simulink model "FSTABSMC"  (R2024b)
settings: Solver=VariableStepAuto  StartTime=0.0  StopTime=20  RelTol=1e-3
settings Model: Creator=amlak  LastModifiedBy=amlak

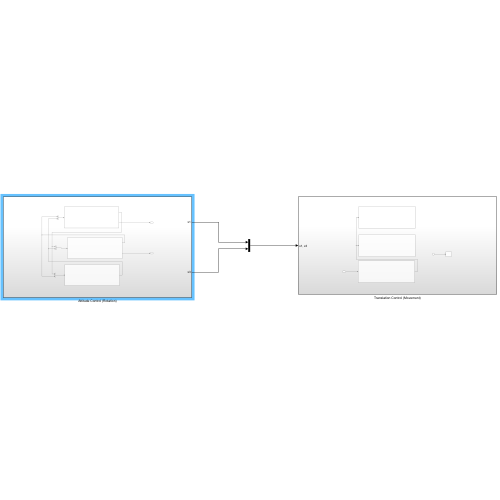
[thumbnail: Simulink's stored preview of the top-level diagram]
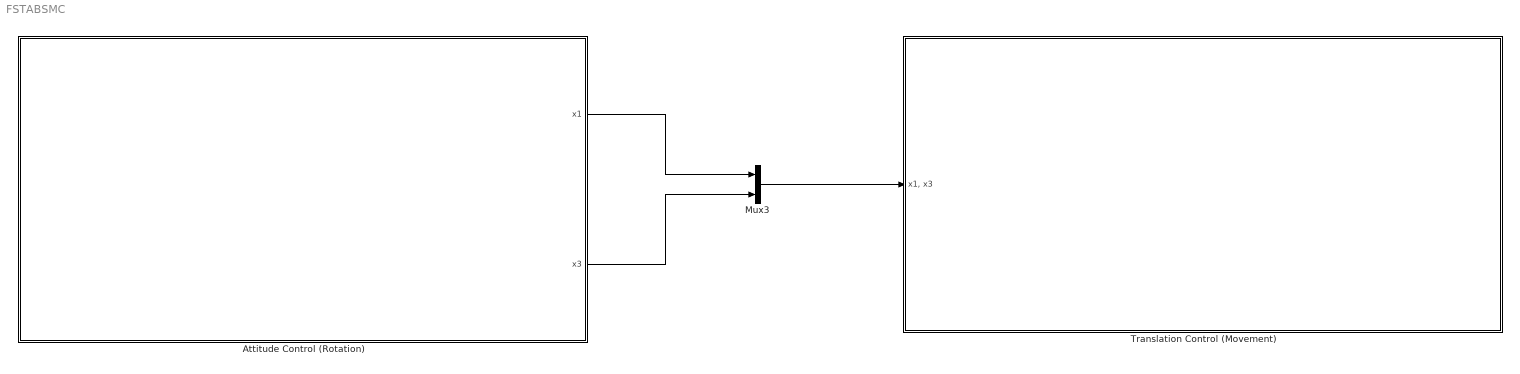
== system FSTABSMC ==
  Attitude Control (Rotation) : Subsystem
  Mux3 : Mux  Inputs=2
  Translation Control (Movement) : Subsystem
  wires:
  Attitude Control (Rotation)/1(x1) -> Mux3/1
  Attitude Control (Rotation)/2(x3) -> Mux3/2
  Mux3/1 -> Translation Control (Movement)/1("x1, x3")

== system FSTABSMC/Attitude Control (Rotation) ==
  Mux : Mux  Inputs=2
  Mux1 : Mux  Inputs=2
  Mux2 : Mux  Inputs=2
  PITCH Controller : Subsystem
  "ROLL Controller " : Subsystem
  YAW Controller : Subsystem
  x1 : Outport
  x3 : Outport  Port=2
  wires:
  YAW Controller/1(x6) -> Mux1/2, Mux/2
  PITCH Controller/1(x4) -> Mux/1, Mux2/2
  "ROLL Controller "/1(x2) -> Mux2/1, Mux1/1
  PITCH Controller/2(x3) -> x3/1
  Mux1/1 -> PITCH Controller/1(In1)
  Mux2/1 -> YAW Controller/1(In1)
  Mux/1 -> "ROLL Controller "/1(In1)
  "ROLL Controller "/2(x1) -> x1/1

== system FSTABSMC/Translation Control (Movement) ==
  "x1, x3" : Inport
  Clock : Clock
      settings: Decimation=20
  To Workspace1 : ToWorkspace  VariableName=t  SampleTime=-1
      settings: Save2DSignal=2-D array (concatenate along first dimension)
  X Trajectory Controller : Subsystem
  Y Trajectory Controller : Subsystem
  "Z Trajectory Controller " : Subsystem
  wires:
  "Z Trajectory Controller "/1(U1) -> X Trajectory Controller/1(U1), Y Trajectory Controller/1(U1)
  "x1, x3"/1 -> "Z Trajectory Controller "/1("x1, x3")
  Clock/1 -> To Workspace1/1

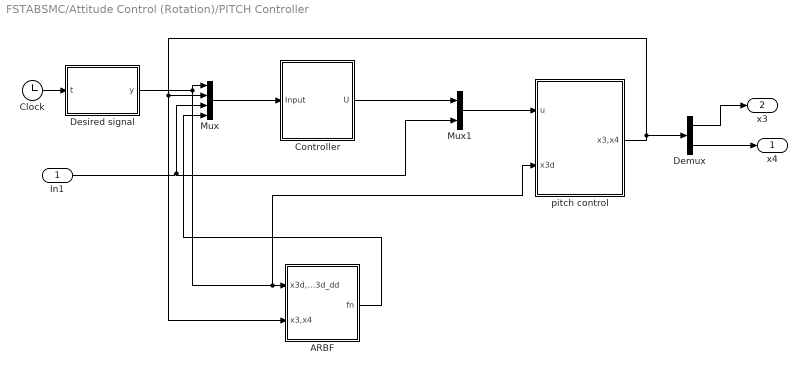
== system FSTABSMC/Attitude Control (Rotation)/PITCH Controller ==
  In1 : Inport
  ARBF : Subsystem
  Clock : Clock
      settings: Decimation=20
  Controller : Subsystem
  Demux : Demux  Outputs=2
  Desired signal : MATLAB Function  TreatAsAtomicUnit=on
  Mux : Mux
  Mux1 : Mux  Inputs=2
  pitch control : Subsystem
  x4 : Outport
  x3 : Outport  Port=2
  wires:
  Desired signal/1(y) -> pitch control/2(x3d), ARBF/1("x3d, x3d_dot, x3d_dd"), Mux/1
  Clock/1 -> Desired signal/1(t)
  pitch control/1(x3,x4) -> Demux/1, ARBF/2(x3,x4), Mux/2
  In1/1 -> Mux/3, Mux1/2
  Mux/1 -> Controller/1(Input)
  Controller/1(U) -> Mux1/1
  Mux1/1 -> pitch control/1(u)
  ARBF/1(fn) -> Mux/4
  Demux/2 -> x4/1
  Demux/1 -> x3/1

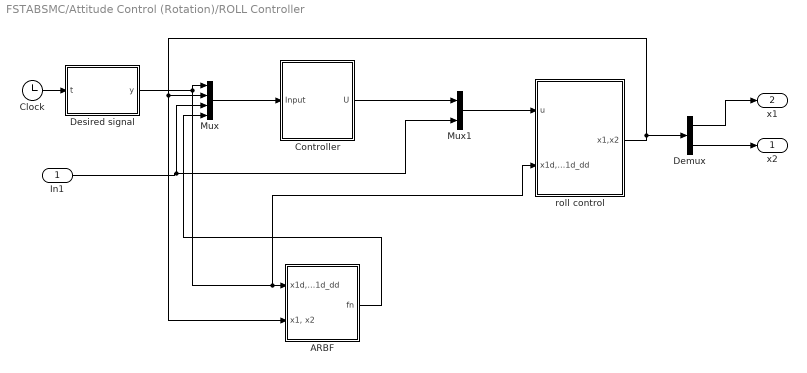
== system FSTABSMC/Attitude Control (Rotation)/ROLL Controller  ==
  In1 : Inport
  ARBF : Subsystem
  Clock : Clock
      settings: Decimation=20
  Controller : Subsystem
  Demux : Demux  Outputs=2
  Desired signal : MATLAB Function  TreatAsAtomicUnit=on
  Mux : Mux
  Mux1 : Mux  Inputs=2
  roll control : Subsystem
  x2 : Outport
  x1 : Outport  Port=2
  wires:
  Desired signal/1(y) -> roll control/2("x1d, x1d_d, x1d_dd"), ARBF/1("x1d, x1d_d, x1d_dd"), Mux/1
  Clock/1 -> Desired signal/1(t)
  roll control/1(x1,x2) -> Demux/1, ARBF/2("x1, x2"), Mux/2
  In1/1 -> Mux1/2, Mux/3
  Mux/1 -> Controller/1(Input)
  Controller/1(U) -> Mux1/1
  Mux1/1 -> roll control/1(u)
  ARBF/1(fn) -> Mux/4
  Demux/2 -> x2/1
  Demux/1 -> x1/1

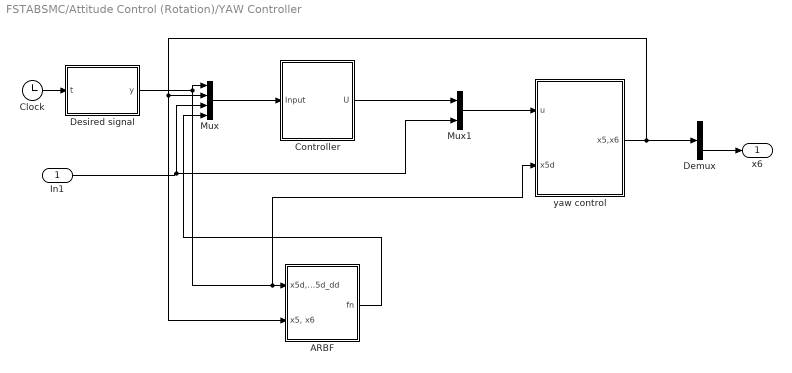
== system FSTABSMC/Attitude Control (Rotation)/YAW Controller ==
  In1 : Inport
  ARBF : Subsystem
  Clock : Clock
      settings: Decimation=20
  Controller : Subsystem
  Demux : Demux  Outputs=2
  Desired signal : MATLAB Function  TreatAsAtomicUnit=on
  Mux : Mux
  Mux1 : Mux  Inputs=2
  yaw control : Subsystem
  x6 : Outport
  wires:
  Desired signal/1(y) -> yaw control/2(x5d), ARBF/1("x5d, x5d_d, x5d_dd"), Mux/1
  Clock/1 -> Desired signal/1(t)
  yaw control/1(x5,x6) -> Demux/1, ARBF/2("x5, x6"), Mux/2
  In1/1 -> Mux1/2, Mux/3
  Mux/1 -> Controller/1(Input)
  Controller/1(U) -> Mux1/1
  Mux1/1 -> yaw control/1(u)
  ARBF/1(fn) -> Mux/4
  Demux/2 -> x6/1

== system FSTABSMC/Translation Control (Movement)/X Trajectory Controller ==
  U1 : Inport
  ARBF : Subsystem
  Clock : Clock
      settings: Decimation=20
  Controller : Subsystem
  Desired signal : MATLAB Function  TreatAsAtomicUnit=on
  Mux : Mux
  Mux1 : Mux  Inputs=2
  x-axis control : Subsystem
  wires:
  Desired signal/1(y) -> x-axis control/2(x7d), ARBF/1("x7d, x7d_d, x7d_dd"), Mux/1
  Clock/1 -> Desired signal/1(t)
  x-axis control/1("x7, x8") -> ARBF/2(x7,x8), Mux/2
  U1/1 -> Mux1/2, Mux/3
  Mux/1 -> Controller/1(Input)
  Controller/1(U) -> Mux1/1
  Mux1/1 -> x-axis control/1(u)
  ARBF/1(fn) -> Mux/4

== system FSTABSMC/Translation Control (Movement)/Y Trajectory Controller ==
  U1 : Inport
  ARBF : Subsystem
  Clock : Clock
      settings: Decimation=20
  Controller : Subsystem
  Desired signal : MATLAB Function  TreatAsAtomicUnit=on
  Mux : Mux
  Mux1 : Mux  Inputs=2
  x-axis control : Subsystem
  wires:
  Desired signal/1(y) -> x-axis control/2(x9d), ARBF/1("x9d, x9d_d, x9d_dd"), Mux/1
  Clock/1 -> Desired signal/1(t)
  x-axis control/1("x9, x10") -> ARBF/2("x9, x10"), Mux/2
  U1/1 -> Mux1/2, Mux/3
  Mux/1 -> Controller/1(Input)
  Controller/1(U) -> Mux1/1
  Mux1/1 -> x-axis control/1(u)
  ARBF/1(fn) -> Mux/4

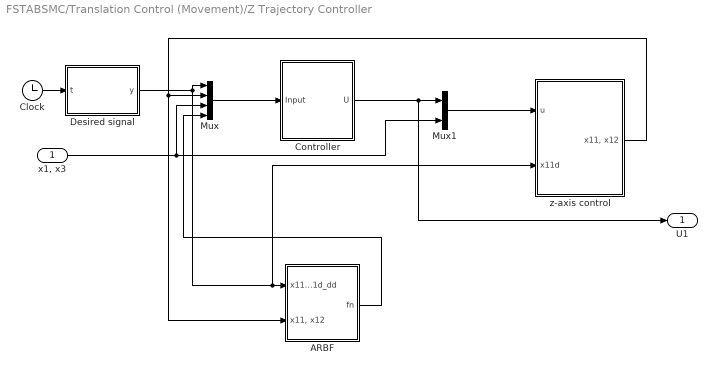
== system FSTABSMC/Translation Control (Movement)/Z Trajectory Controller  ==
  "x1, x3" : Inport
  ARBF : Subsystem
  Clock : Clock
      settings: Decimation=20
  Controller : Subsystem
  Desired signal : MATLAB Function  TreatAsAtomicUnit=on
  Mux : Mux
  Mux1 : Mux  Inputs=2
  z-axis control : Subsystem
  U1 : Outport
  wires:
  Desired signal/1(y) -> z-axis control/2(x11d), ARBF/1("x11d, x11d_d, x11d_dd"), Mux/1
  Clock/1 -> Desired signal/1(t)
  z-axis control/1("x11, x12") -> ARBF/2("x11, x12"), Mux/2
  "x1, x3"/1 -> Mux1/2, Mux/3
  Mux/1 -> Controller/1(Input)
  Controller/1(U) -> Mux1/1, U1/1
  Mux1/1 -> z-axis control/1(u)
  ARBF/1(fn) -> Mux/4

== system FSTABSMC/Attitude Control (Rotation)/PITCH Controller/ARBF ==
  "x3d, x3d_dot, x3d_dd" : Inport
  x3,x4 : Inport  Port=2
  ARBF : MATLABFcn  MATLABFcn=ARBF_theta  OutputDimensions=20
  Demux : Demux  Outputs=[1 19]
  Integrator1 : Integrator
  Mux : Mux  Inputs=3
  fn : Outport
  wires:
  ARBF/1 -> Demux/1
  Mux/1 -> ARBF/1
  x3,x4/1 -> Mux/2
  Demux/2 -> Integrator1/1
  Integrator1/1 -> Mux/3
  "x3d, x3d_dot, x3d_dd"/1 -> Mux/1
  Demux/1 -> fn/1

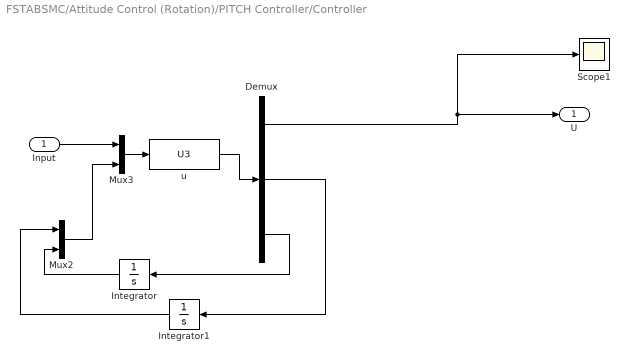
== system FSTABSMC/Attitude Control (Rotation)/PITCH Controller/Controller ==
  Input : Inport
  Demux : Demux  Outputs=3
  Integrator : Integrator
  Integrator1 : Integrator
  Mux2 : Mux  Inputs=2
  Mux3 : Mux  Inputs=2
  Scope1 : Scope
  u : MATLABFcn  MATLABFcn=U3  OutputDimensions=3
  U : Outport
  wires:
  u/1 -> Demux/1
  Demux/1 -> Scope1/1, U/1
  Demux/2 -> Integrator1/1
  Demux/3 -> Integrator/1
  Mux2/1 -> Mux3/2
  Mux3/1 -> u/1
  Input/1 -> Mux3/1
  Integrator/1 -> Mux2/2
  Integrator1/1 -> Mux2/1

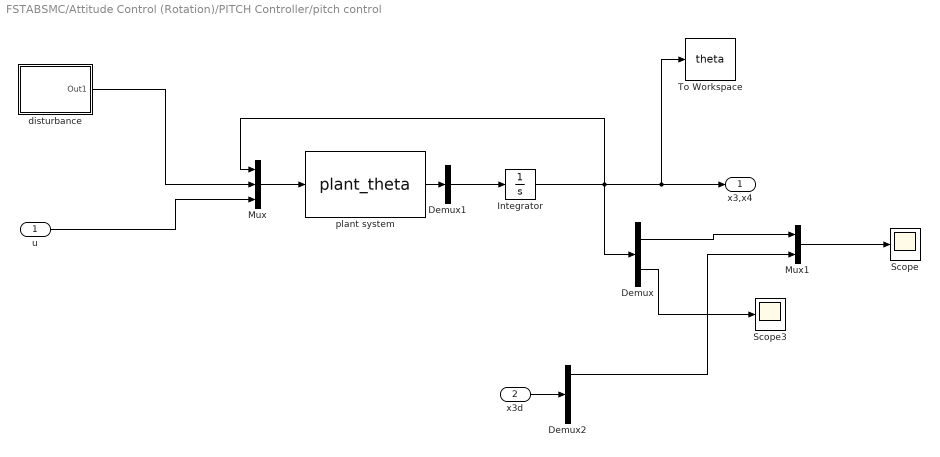
== system FSTABSMC/Attitude Control (Rotation)/PITCH Controller/pitch control ==
  u : Inport
  x3d : Inport  Port=2
  Demux : Demux  Outputs=2
  Demux1 : Demux  Outputs=1
  Demux2 : Demux  Outputs=3
  Integrator : Integrator  InitialCondition=[3;0]
  Mux : Mux  Inputs=3
  Mux1 : Mux  Inputs=2
  Scope : Scope
  Scope3 : Scope
  To Workspace : ToWorkspace  VariableName=theta  SampleTime=-1
      settings: Save2DSignal=2-D array (concatenate along first dimension)
  disturbance : Subsystem
  plant system : MATLABFcn  MATLABFcn=plant_theta  OutputDimensions=2
  x3,x4 : Outport
  wires:
  Mux/1 -> plant system/1
  Integrator/1 -> Mux/1, Demux/1, To Workspace/1, x3,x4/1
  u/1 -> Mux/3
  disturbance/1(Out1) -> Mux/2
  Demux/1 -> Mux1/1
  Mux1/1 -> Scope/1
  Demux/2 -> Scope3/1
  plant system/1 -> Demux1/1
  Demux1/1 -> Integrator/1
  x3d/1 -> Demux2/1
  Demux2/1 -> Mux1/2

== system FSTABSMC/Attitude Control (Rotation)/ROLL Controller /ARBF ==
  "x1d, x1d_d, x1d_dd" : Inport
  "x1, x2" : Inport  Port=2
  ARBF : MATLABFcn  MATLABFcn=ARBF_phi  OutputDimensions=20
  Demux : Demux  Outputs=[1 19]
  Integrator1 : Integrator
  Mux : Mux  Inputs=3
  fn : Outport
  wires:
  ARBF/1 -> Demux/1
  Mux/1 -> ARBF/1
  "x1, x2"/1 -> Mux/2
  Demux/2 -> Integrator1/1
  Integrator1/1 -> Mux/3
  "x1d, x1d_d, x1d_dd"/1 -> Mux/1
  Demux/1 -> fn/1

== system FSTABSMC/Attitude Control (Rotation)/ROLL Controller /Controller ==
  Input : Inport
  Demux : Demux  Outputs=3
  Integrator : Integrator
  Integrator1 : Integrator
  Mux2 : Mux  Inputs=2
  Mux3 : Mux  Inputs=2
  Scope1 : Scope
  u : MATLABFcn  MATLABFcn=U2  OutputDimensions=3
  U : Outport
  wires:
  u/1 -> Demux/1
  Demux/1 -> Scope1/1, U/1
  Demux/2 -> Integrator1/1
  Demux/3 -> Integrator/1
  Mux2/1 -> Mux3/2
  Mux3/1 -> u/1
  Input/1 -> Mux3/1
  Integrator/1 -> Mux2/2
  Integrator1/1 -> Mux2/1

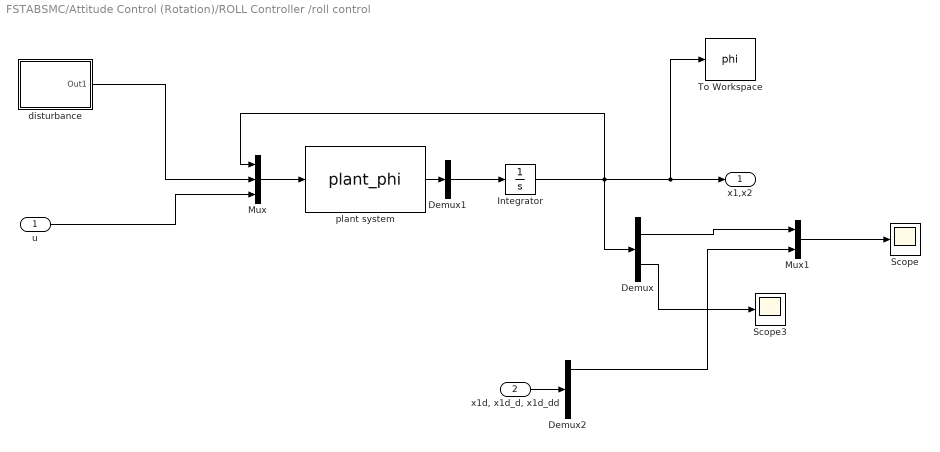
== system FSTABSMC/Attitude Control (Rotation)/ROLL Controller /roll control ==
  u : Inport
  "x1d, x1d_d, x1d_dd" : Inport  Port=2
  Demux : Demux  Outputs=2
  Demux1 : Demux  Outputs=1
  Demux2 : Demux  Outputs=3
  Integrator : Integrator  InitialCondition=[2;0]
  Mux : Mux  Inputs=3
  Mux1 : Mux  Inputs=2
  Scope : Scope
  Scope3 : Scope
  To Workspace : ToWorkspace  VariableName=phi  SampleTime=-1
      settings: Save2DSignal=2-D array (concatenate along first dimension)
  disturbance : Subsystem
  plant system : MATLABFcn  MATLABFcn=plant_phi  OutputDimensions=2
  x1,x2 : Outport
  wires:
  Mux/1 -> plant system/1
  Integrator/1 -> Mux/1, Demux/1, To Workspace/1, x1,x2/1
  u/1 -> Mux/3
  disturbance/1(Out1) -> Mux/2
  Demux/1 -> Mux1/1
  Mux1/1 -> Scope/1
  Demux/2 -> Scope3/1
  plant system/1 -> Demux1/1
  Demux1/1 -> Integrator/1
  "x1d, x1d_d, x1d_dd"/1 -> Demux2/1
  Demux2/1 -> Mux1/2

== system FSTABSMC/Attitude Control (Rotation)/YAW Controller/ARBF ==
  "x5d, x5d_d, x5d_dd" : Inport
  "x5, x6" : Inport  Port=2
  ARBF : MATLABFcn  MATLABFcn=ARBF_psi  OutputDimensions=20
  Demux : Demux  Outputs=[1 19]
  Integrator1 : Integrator
  Mux : Mux  Inputs=3
  fn : Outport
  wires:
  ARBF/1 -> Demux/1
  Mux/1 -> ARBF/1
  "x5, x6"/1 -> Mux/2
  Demux/2 -> Integrator1/1
  Integrator1/1 -> Mux/3
  "x5d, x5d_d, x5d_dd"/1 -> Mux/1
  Demux/1 -> fn/1

== system FSTABSMC/Attitude Control (Rotation)/YAW Controller/Controller ==
  Input : Inport
  Demux : Demux  Outputs=3
  Integrator : Integrator
  Integrator1 : Integrator
  Mux2 : Mux  Inputs=2
  Mux3 : Mux  Inputs=2
  Scope1 : Scope
  u : MATLABFcn  MATLABFcn=U4  OutputDimensions=3
  U : Outport
  wires:
  u/1 -> Demux/1
  Demux/1 -> Scope1/1, U/1
  Demux/2 -> Integrator1/1
  Demux/3 -> Integrator/1
  Mux2/1 -> Mux3/2
  Mux3/1 -> u/1
  Input/1 -> Mux3/1
  Integrator/1 -> Mux2/2
  Integrator1/1 -> Mux2/1

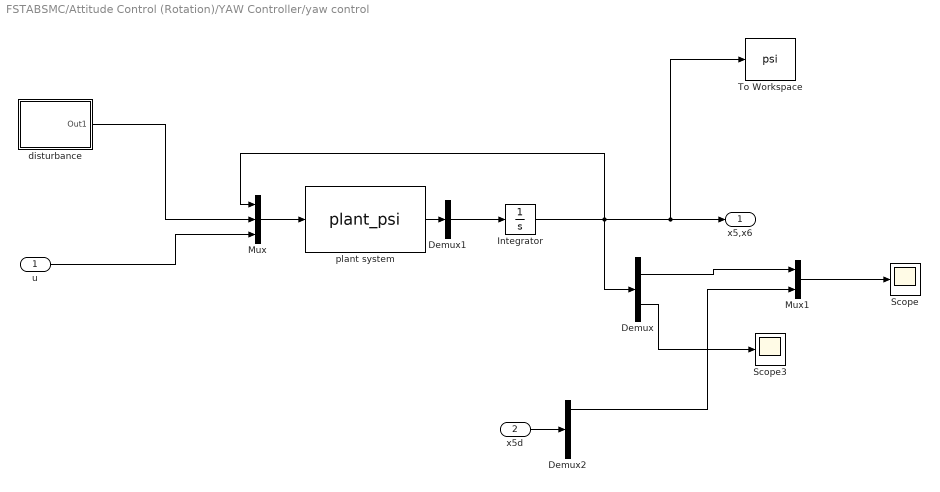
== system FSTABSMC/Attitude Control (Rotation)/YAW Controller/yaw control ==
  u : Inport
  x5d : Inport  Port=2
  Demux : Demux  Outputs=2
  Demux1 : Demux  Outputs=1
  Demux2 : Demux  Outputs=3
  Integrator : Integrator  InitialCondition=[1;0]
  Mux : Mux  Inputs=3
  Mux1 : Mux  Inputs=2
  Scope : Scope
  Scope3 : Scope
  To Workspace : ToWorkspace  VariableName=psi  SampleTime=-1
      settings: Save2DSignal=2-D array (concatenate along first dimension)
  disturbance : Subsystem
  plant system : MATLABFcn  MATLABFcn=plant_psi  OutputDimensions=2
  x5,x6 : Outport
  wires:
  Mux/1 -> plant system/1
  Integrator/1 -> Mux/1, Demux/1, To Workspace/1, x5,x6/1
  u/1 -> Mux/3
  disturbance/1(Out1) -> Mux/2
  Demux/1 -> Mux1/1
  Mux1/1 -> Scope/1
  Demux/2 -> Scope3/1
  plant system/1 -> Demux1/1
  Demux1/1 -> Integrator/1
  x5d/1 -> Demux2/1
  Demux2/1 -> Mux1/2

== system FSTABSMC/Translation Control (Movement)/X Trajectory Controller/ARBF ==
  "x7d, x7d_d, x7d_dd" : Inport
  x7,x8 : Inport  Port=2
  ARBF : MATLABFcn  MATLABFcn=ARBF_x  OutputDimensions=20
  Demux : Demux  Outputs=[1 19]
  Integrator1 : Integrator
  Mux : Mux  Inputs=3
  fn : Outport
  wires:
  ARBF/1 -> Demux/1
  Mux/1 -> ARBF/1
  x7,x8/1 -> Mux/2
  Demux/2 -> Integrator1/1
  Integrator1/1 -> Mux/3
  "x7d, x7d_d, x7d_dd"/1 -> Mux/1
  Demux/1 -> fn/1

== system FSTABSMC/Translation Control (Movement)/X Trajectory Controller/Controller ==
  Input : Inport
  Demux : Demux  Outputs=3
  Integrator : Integrator
  Integrator1 : Integrator
  Mux2 : Mux  Inputs=2
  Mux3 : Mux  Inputs=2
  Scope1 : Scope
  u : MATLABFcn  MATLABFcn=Ux  OutputDimensions=3
  U : Outport
  wires:
  u/1 -> Demux/1
  Demux/1 -> Scope1/1, U/1
  Demux/2 -> Integrator1/1
  Demux/3 -> Integrator/1
  Mux2/1 -> Mux3/2
  Mux3/1 -> u/1
  Input/1 -> Mux3/1
  Integrator/1 -> Mux2/2
  Integrator1/1 -> Mux2/1

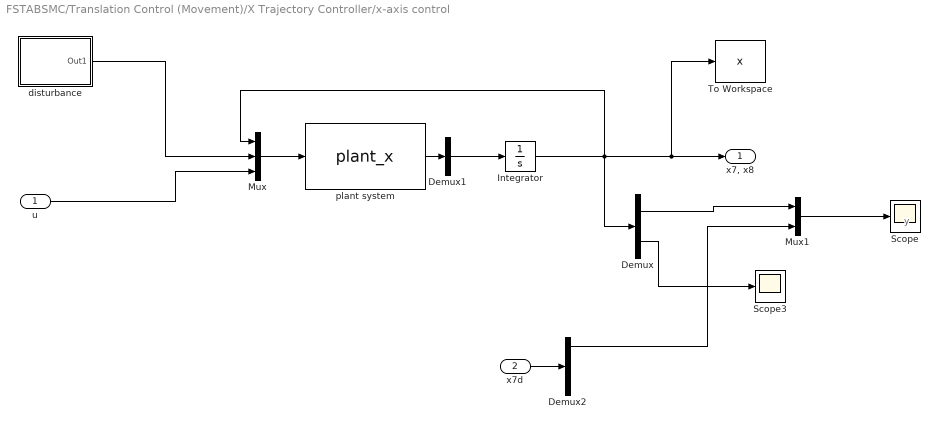
== system FSTABSMC/Translation Control (Movement)/X Trajectory Controller/x-axis control ==
  note: y
  u : Inport
  x7d : Inport  Port=2
  Demux : Demux  Outputs=2
  Demux1 : Demux  Outputs=1
  Demux2 : Demux  Outputs=3
  Integrator : Integrator  InitialCondition=[1;0]
  Mux : Mux  Inputs=3
  Mux1 : Mux  Inputs=2
  Scope : Scope
  Scope3 : Scope
  To Workspace : ToWorkspace  VariableName=x  SampleTime=-1
      settings: Save2DSignal=2-D array (concatenate along first dimension)
  disturbance : Subsystem
  plant system : MATLABFcn  MATLABFcn=plant_x  OutputDimensions=2
  "x7, x8" : Outport
  wires:
  Mux/1 -> plant system/1
  Integrator/1 -> Mux/1, Demux/1, To Workspace/1, "x7, x8"/1
  u/1 -> Mux/3
  disturbance/1(Out1) -> Mux/2
  Demux/1 -> Mux1/1
  Mux1/1 -> Scope/1
  Demux/2 -> Scope3/1
  plant system/1 -> Demux1/1
  Demux1/1 -> Integrator/1
  x7d/1 -> Demux2/1
  Demux2/1 -> Mux1/2

== system FSTABSMC/Translation Control (Movement)/Y Trajectory Controller/ARBF ==
  "x9d, x9d_d, x9d_dd" : Inport
  "x9, x10" : Inport  Port=2
  ARBF : MATLABFcn  MATLABFcn=ARBF_y  OutputDimensions=20
  Demux : Demux  Outputs=[1 19]
  Integrator1 : Integrator
  Mux : Mux  Inputs=3
  fn : Outport
  wires:
  ARBF/1 -> Demux/1
  Mux/1 -> ARBF/1
  "x9, x10"/1 -> Mux/2
  Demux/2 -> Integrator1/1
  Integrator1/1 -> Mux/3
  "x9d, x9d_d, x9d_dd"/1 -> Mux/1
  Demux/1 -> fn/1

== system FSTABSMC/Translation Control (Movement)/Y Trajectory Controller/Controller ==
  Input : Inport
  Demux : Demux  Outputs=3
  Integrator : Integrator
  Integrator1 : Integrator
  Mux2 : Mux  Inputs=2
  Mux3 : Mux  Inputs=2
  Scope1 : Scope
  u : MATLABFcn  MATLABFcn=Uy  OutputDimensions=3
  U : Outport
  wires:
  u/1 -> Demux/1
  Demux/1 -> Scope1/1, U/1
  Demux/2 -> Integrator1/1
  Demux/3 -> Integrator/1
  Mux2/1 -> Mux3/2
  Mux3/1 -> u/1
  Input/1 -> Mux3/1
  Integrator/1 -> Mux2/2
  Integrator1/1 -> Mux2/1

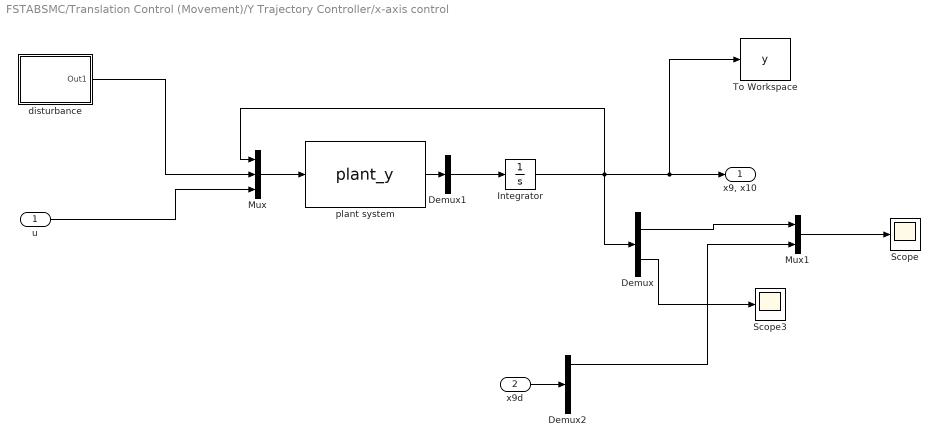
== system FSTABSMC/Translation Control (Movement)/Y Trajectory Controller/x-axis control ==
  u : Inport
  x9d : Inport  Port=2
  Demux : Demux  Outputs=2
  Demux1 : Demux  Outputs=1
  Demux2 : Demux  Outputs=3
  Integrator : Integrator  InitialCondition=[1;0]
  Mux : Mux  Inputs=3
  Mux1 : Mux  Inputs=2
  Scope : Scope
  Scope3 : Scope
  To Workspace : ToWorkspace  VariableName=y  SampleTime=-1
      settings: Save2DSignal=2-D array (concatenate along first dimension)
  disturbance : Subsystem
  plant system : MATLABFcn  MATLABFcn=plant_y  OutputDimensions=2
  "x9, x10" : Outport
  wires:
  Mux/1 -> plant system/1
  Integrator/1 -> Mux/1, Demux/1, To Workspace/1, "x9, x10"/1
  u/1 -> Mux/3
  disturbance/1(Out1) -> Mux/2
  Demux/1 -> Mux1/1
  Mux1/1 -> Scope/1
  Demux/2 -> Scope3/1
  plant system/1 -> Demux1/1
  Demux1/1 -> Integrator/1
  x9d/1 -> Demux2/1
  Demux2/1 -> Mux1/2

== system FSTABSMC/Translation Control (Movement)/Z Trajectory Controller /ARBF ==
  "x11d, x11d_d, x11d_dd" : Inport
  "x11, x12" : Inport  Port=2
  ARBF : MATLABFcn  MATLABFcn=ARBF_z  OutputDimensions=20
  Demux : Demux  Outputs=[1 19]
  Integrator1 : Integrator
  Mux : Mux  Inputs=3
  fn : Outport
  wires:
  ARBF/1 -> Demux/1
  Mux/1 -> ARBF/1
  "x11, x12"/1 -> Mux/2
  Demux/2 -> Integrator1/1
  Integrator1/1 -> Mux/3
  "x11d, x11d_d, x11d_dd"/1 -> Mux/1
  Demux/1 -> fn/1

== system FSTABSMC/Translation Control (Movement)/Z Trajectory Controller /Controller ==
  Input : Inport
  Demux : Demux  Outputs=3
  Integrator : Integrator
  Integrator1 : Integrator
  Mux2 : Mux  Inputs=2
  Mux3 : Mux  Inputs=2
  Scope1 : Scope
  u : MATLABFcn  MATLABFcn=U1  OutputDimensions=3
  U : Outport
  wires:
  u/1 -> Demux/1
  Demux/1 -> Scope1/1, U/1
  Demux/2 -> Integrator1/1
  Demux/3 -> Integrator/1
  Mux2/1 -> Mux3/2
  Mux3/1 -> u/1
  Input/1 -> Mux3/1
  Integrator/1 -> Mux2/2
  Integrator1/1 -> Mux2/1

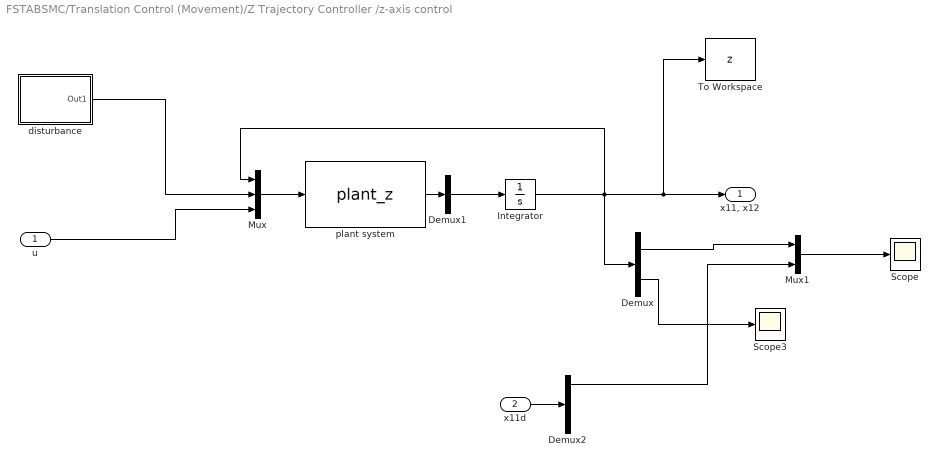
== system FSTABSMC/Translation Control (Movement)/Z Trajectory Controller /z-axis control ==
  u : Inport
  x11d : Inport  Port=2
  Demux : Demux  Outputs=2
  Demux1 : Demux  Outputs=1
  Demux2 : Demux  Outputs=3
  Integrator : Integrator  InitialCondition=[1;0]
  Mux : Mux  Inputs=3
  Mux1 : Mux  Inputs=2
  Scope : Scope
  Scope3 : Scope
  To Workspace : ToWorkspace  VariableName=z  SampleTime=-1
      settings: Save2DSignal=2-D array (concatenate along first dimension)
  disturbance : Subsystem
  plant system : MATLABFcn  MATLABFcn=plant_z  OutputDimensions=2
  "x11, x12" : Outport
  wires:
  Mux/1 -> plant system/1
  Integrator/1 -> Mux/1, Demux/1, To Workspace/1, "x11, x12"/1
  u/1 -> Mux/3
  disturbance/1(Out1) -> Mux/2
  Demux/1 -> Mux1/1
  Mux1/1 -> Scope/1
  Demux/2 -> Scope3/1
  plant system/1 -> Demux1/1
  Demux1/1 -> Integrator/1
  x11d/1 -> Demux2/1
  Demux2/1 -> Mux1/2

== system FSTABSMC/Attitude Control (Rotation)/PITCH Controller/pitch control/disturbance ==
  Gain2 : Gain  Gain=10
  Scope : Scope
  d2 : Sin  Amplitude=3  SampleTime=0
  Out1 : Outport
  wires:
  d2/1 -> Gain2/1
  Gain2/1 -> Out1/1, Scope/1

== system FSTABSMC/Attitude Control (Rotation)/ROLL Controller /roll control/disturbance ==
  Gain2 : Gain  Gain=10
  Scope : Scope
  d2 : Sin  Amplitude=3  SampleTime=0
  Out1 : Outport
  wires:
  d2/1 -> Gain2/1
  Gain2/1 -> Out1/1, Scope/1

== system FSTABSMC/Attitude Control (Rotation)/YAW Controller/yaw control/disturbance ==
  Gain2 : Gain  Gain=10
  Scope : Scope
  d2 : Sin  Amplitude=3  SampleTime=0
  Out1 : Outport
  wires:
  d2/1 -> Gain2/1
  Gain2/1 -> Out1/1, Scope/1

== system FSTABSMC/Translation Control (Movement)/X Trajectory Controller/x-axis control/disturbance ==
  Gain2 : Gain  Gain=10
  Scope : Scope
  d2 : Sin  Amplitude=4  SampleTime=0
  Out1 : Outport
  wires:
  d2/1 -> Gain2/1
  Gain2/1 -> Out1/1, Scope/1

== system FSTABSMC/Translation Control (Movement)/Y Trajectory Controller/x-axis control/disturbance ==
  Gain2 : Gain  Gain=10
  Scope : Scope
  d2 : Sin  Amplitude=4  SampleTime=0
  Out1 : Outport
  wires:
  d2/1 -> Gain2/1
  Gain2/1 -> Out1/1, Scope/1

== system FSTABSMC/Translation Control (Movement)/Z Trajectory Controller /z-axis control/disturbance ==
  Gain2 : Gain  Gain=10
  Scope : Scope
  d2 : Sin  Amplitude=4  SampleTime=0
  Out1 : Outport
  wires:
  d2/1 -> Gain2/1
  Gain2/1 -> Out1/1, Scope/1

== matlab function FSTABSMC/Translation Control (Movement)/X Trajectory Controller/Desired signal ==
  data: t input; y output
function y = fcn(t)

x7d = (3 + cos(5*t))*cos(t);

x7d_d = -sin(t)*(3+cos(5*t)) + cos(t)*(-5*sin(5*t));

x7d_dd = -cos(t)*(3+cos(5*t)) + sin(t)*(5*sin(5*t)) - sin(t)*(-5*sin(5*t)) + cos(t)*(-25*cos(5*t));
y = [x7d, x7d_d, x7d_dd]';

== matlab function FSTABSMC/Attitude Control (Rotation)/PITCH Controller/Desired signal ==
  data: t input; y output
function y = fcn(t)

x3d = cos(t);

x3d_d = -sin(t);

x3d_dd = -cos(t);
y = [x3d, x3d_d, x3d_dd]';

== matlab function FSTABSMC/Attitude Control (Rotation)/YAW Controller/Desired signal ==
  data: t input; y output
function y = fcn(t)

x1d = 0.1*t;

x1d_d = 0.1;

x1d_dd = 0;
y = [x1d, x1d_d, x1d_dd]';

== matlab function FSTABSMC/Translation Control (Movement)/Y Trajectory Controller/Desired signal ==
  data: t input; y output
function y = fcn(t)

x9d = (3 + cos(5*t))*sin(t);

x9d_d = cos(t)*(3+cos(5*t)) + sin(t)*(-5*sin(5*t));

x9d_dd = -sin(t)*(3+cos(5*t)) + cos(t)*(5*sin(5*t)) + cos(t)*(-5*sin(5*t)) + sin(t)*(-25*cos(5*t));
y = [x9d, x9d_d, x9d_dd]';

== matlab function FSTABSMC/Translation Control (Movement)/Z Trajectory Controller /Desired signal ==
  data: t input; y output
function y = fcn(t)

x11d = sin(5*t);

x11d_d = 5*cos(5*t);

x11d_dd = -25*sin(5*t);
y = [x11d, x11d_d, x11d_dd]';

== matlab function FSTABSMC/Attitude Control (Rotation)/ROLL Controller /Desired signal ==
  data: t input; y output
function y = fcn(t)

x1d = sin(t);

x1d_d = cos(t);

x1d_dd = -sin(t);
y = [x1d, x1d_d, x1d_dd]';
